simulink model "modelo_a"  (R2026a)
settings: Solver=ode4  StopTime=t_final  FixedStep=dt
values from neighbouring files (symbols this model uses):
  T = 1    [init.m]
  theta = 5    [init.m]
settings Model: Creator=honda  LastModifiedBy=honda

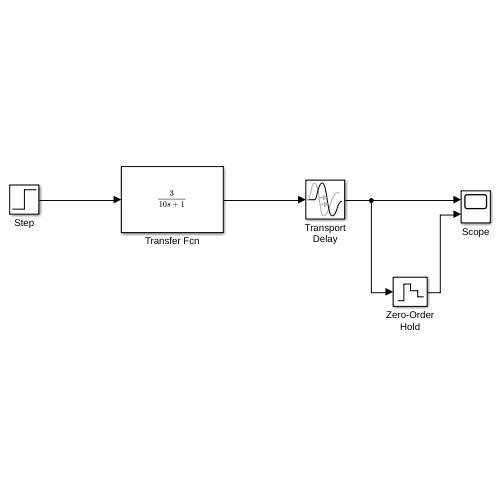
[thumbnail: Simulink's stored preview of the top-level diagram]
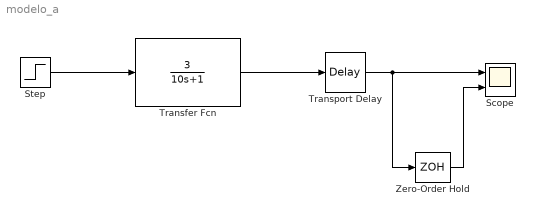
== system modelo_a ==
  Scope : Scope  NumInputPorts=2
      settings: ActiveDisplayYMinimum=-0.032424926878626928  ActiveDisplayYMaximum=0.29182434190764239  DataLoggingVariableName=dados_a
  Step : Step  Time=0  FinalValue=u0  SampleTime=0
  Transfer Fcn : TransferFcn  Numerator=[3]  Denominator=[10 1]
  Transport Delay : TransportDelay  DelayTime=theta
  Zero-Order Hold : ZeroOrderHold  SampleTime=T
  wires:
  Step/1 -> Transfer Fcn/1
  Transfer Fcn/1 -> Transport Delay/1
  Transport Delay/1 -> Zero-Order Hold/1, Scope/1
  Zero-Order Hold/1 -> Scope/2
